simulink model "TireMF62"  (R2026b)
settings: Solver=ode45  StopTime=1
settings Model: DataDictionary=VehicleData.sldd  Creator=Xu Dingyi  LastModifiedBy=29358

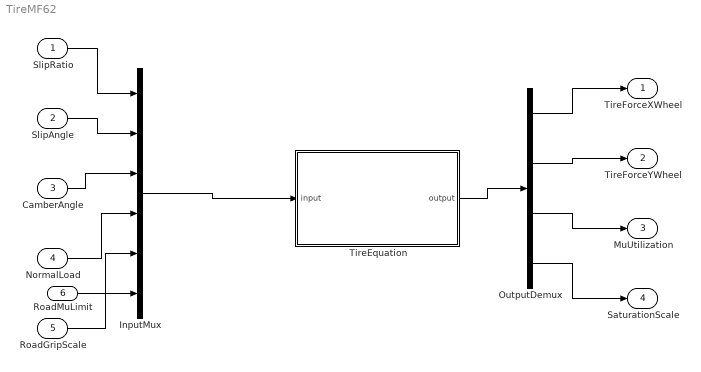
== system TireMF62 ==
  SlipRatio : Inport  PortDimensions=4
  SlipAngle : Inport  Port=2  PortDimensions=4
  CamberAngle : Inport  Port=3  PortDimensions=4
  NormalLoad : Inport  Port=4  PortDimensions=4
  RoadGripScale : Inport  Port=5  PortDimensions=4
  RoadMuLimit : Inport  Port=6  PortDimensions=4
  InputMux : Mux  Inputs=6
  OutputDemux : Demux  Outputs=[4 4 4 4]
  TireEquation : MATLAB Function  TreatAsAtomicUnit=on
  TireForceXWheel : Outport
  TireForceYWheel : Outport  Port=2
  MuUtilization : Outport  Port=3
  SaturationScale : Outport  Port=4
  wires:
  SlipRatio/1 -> InputMux/1
  SlipAngle/1 -> InputMux/2
  CamberAngle/1 -> InputMux/3
  NormalLoad/1 -> InputMux/4
  RoadGripScale/1 -> InputMux/5
  InputMux/1 -> TireEquation/1(input)
  TireEquation/1(output) -> OutputDemux/1
  OutputDemux/1 -> TireForceXWheel/1
  OutputDemux/2 -> TireForceYWheel/1
  OutputDemux/3 -> MuUtilization/1
  OutputDemux/4 -> SaturationScale/1
  RoadMuLimit/1 -> InputMux/6

== matlab function TireMF62/TireEquation ==
  data: input input; output output; TireMFParameters parameter
function output = tireEquation(input, TireMFParameters)
%#codegen
output = evaluateTireMF62Codegen(input, TireMFParameters);
end
